simulink model "systeme_sol_2017a"  (R2017a)
settings: Solver=VariableStepAuto  StartTime=0.0  StopTime=100000  RelTol=1e-3
values from neighbouring files (symbols this model uses):
  A_solar_tank_1 = eval(A_solar_tank)    [Maple_linearization2.m]
  B_solar_tank_1 = eval(B_solar_tank(:,1:2))    [Maple_linearization2.m]
  Bd_solar_tank_1 = eval(B_solar_tank(:,3:5))    [Maple_linearization2.m]
  C_solar_tank_1 = eye(3)    [Maple_linearization2.m]
  D_solar_tank_1 = zeros(3,5)    [Maple_linearization2.m]
  Tcin = 47.5    [Maple_linearization2.m]
  Tcout = 60    [Maple_linearization2.m]
  Ttout = 27.5    [Maple_linearization2.m]
settings Model: Creator=julien  LastModifiedBy=admin
settings DataIOCC: ReturnWorkspaceOutputs=on
settings SFSimCC: SimUseLocalCustomCode=on
settings RTWCC: RTWUseLocalCustomCode=on

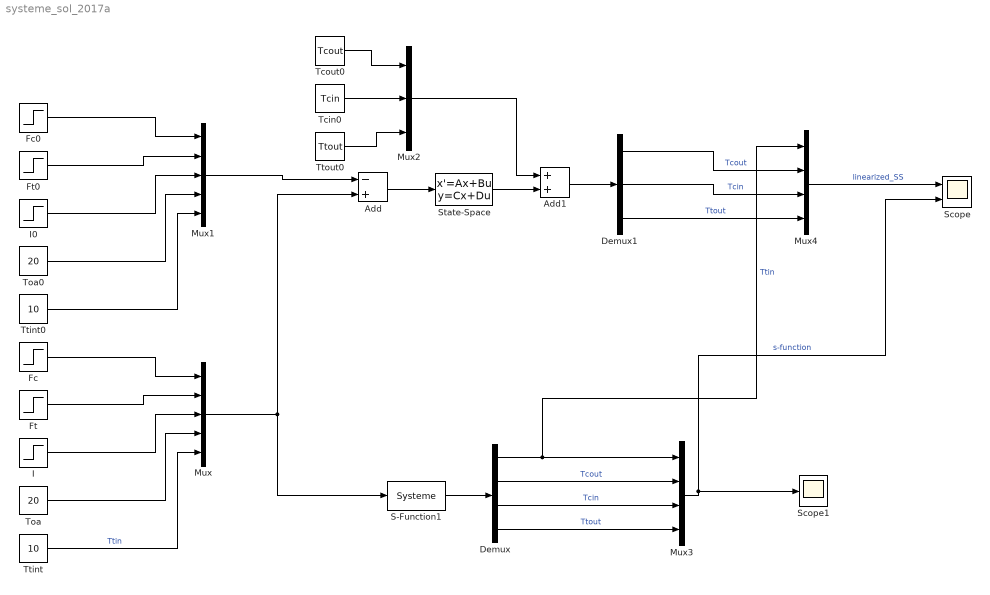
== system systeme_sol_2017a ==
  Add : Sum  Inputs=-+
  Add1 : Sum
  Demux : Demux
  Demux1 : Demux  Outputs=3
  Fc : Step  Time=0  After=1.5e-5  SampleTime=0
  Fc0 : Step  Time=0  After=1.5e-5  SampleTime=0
  Ft : Step  Time=0  After=1e-5  SampleTime=0
  Ft0 : Step  Time=0  After=1e-5  SampleTime=0
  I : Step  Time=50000  Before=1000  After=1000  SampleTime=0
  I0 : Step  Time=0  After=1000  SampleTime=0
  Mux : Mux  Inputs=5
  Mux1 : Mux  Inputs=5
  Mux2 : Mux  Inputs=3
  Mux3 : Mux
  Mux4 : Mux
  S-Function1 : S-Function  FunctionName=Systeme  Parameters=Tcout,Tcin,Ttout  SFunctionDeploymentMode=off  EnableBusSupport=off
  Scope : Scope  NumInputPorts=2
  Scope1 : Scope
  State-Space : StateSpace  A=A_solar_tank_1  B=[B_solar_tank_1 Bd_solar_tank_1]  C=C_solar_tank_1  D=D_solar_tank_1  X0=[0 0 0]
  Tcin0 : Constant  Value=Tcin
  Tcout0 : Constant  Value=Tcout
  Toa : Constant  Value=20
  Toa0 : Constant  Value=20
  Ttint : Constant  Value=10
  Ttint0 : Constant  Value=10
  Ttout0 : Constant  Value=Ttout
  wires:
  Fc/1 -> Mux/1
  Ft/1 -> Mux/2
  I/1 -> Mux/3
  Toa/1 -> Mux/4
  Ttint/1 -> Mux/5  "Ttin"
  Mux/1 -> Add/2, S-Function1/1
  Add/1 -> State-Space/1
  Ttint0/1 -> Mux1/5
  Toa0/1 -> Mux1/4
  I0/1 -> Mux1/3
  Ft0/1 -> Mux1/2
  Fc0/1 -> Mux1/1
  Mux1/1 -> Add/1
  State-Space/1 -> Add1/2
  Tcout0/1 -> Mux2/1
  Tcin0/1 -> Mux2/2
  Ttout0/1 -> Mux2/3
  Mux2/1 -> Add1/1
  S-Function1/1 -> Demux/1
  Mux3/1 -> Scope1/1, Scope/2  "s-function"
  Demux/4 -> Mux3/4  "Ttout"
  Demux/3 -> Mux3/3  "Tcin"
  Demux/2 -> Mux3/2  "Tcout"
  Demux/1 -> Mux4/1, Mux3/1  "Ttin"
  Add1/1 -> Demux1/1
  Demux1/1 -> Mux4/2  "Tcout"
  Demux1/2 -> Mux4/3  "Tcin"
  Demux1/3 -> Mux4/4  "Ttout"
  Mux4/1 -> Scope/1  "linearized_SS"
